simulink model "Jq_cc"  (R2015b)
settings: Solver=FixedStepDiscrete  StartTime=0.0  StopTime=0.01  FixedStep=0.010  RelTol=1e-3
PostLoadFcn:
  | , if any(exist('dsrtsu_mdlpostloadfcn', 'file') == [2, 3, 6]), try dsrtsu_mdlpostloadfcn('Execute', bdroot); catch fprintf('Error in PostLoadFcn (dsrtsu_mdlpostloadfcn) for model "%s":\n %s\n', bdroot, lasterr); end, end,
undefined symbols (not defined in the file or in its folder): DiscIntNeverNeededParam, lData
settings Model: DSRTSU_INTERNAL_RTI_VER=440  DSRTSU_INTERNAL_RTI_TYPE=rti1007  DSRTSU_INTERNAL_RTIFPGA=30  Creator=Mahl  LastModifiedBy=Mayer
settings DataIOCC: SaveFormat=Array
settings OptimizationCC: BlockReduction=off  OptimizeBlockIOStorage=off  BufferReuse=off  GlobalBufferReuse=off  ExpressionFolding=off  ExpressionDepthLimit=2147483647  LocalBlockOutputs=off
settings DebuggingCC: SolverPrmCheckMsg=warning  StateNameClashWarn=warning
settings HardwareCC: ProdBitPerPointer=32  ProdLargestAtomicFloat=None  ProdEndianess=BigEndian  ProdWordSize=32  ProdHWDeviceType=Generic->Custom  TargetIntDivRoundTo=Zero  TargetEndianess=BigEndian  TargetHWDeviceType=Generic->Custom
settings RTWCC: SystemTargetFile=rti1103.tlc  MakeCommand=make_rti  TemplateMakefile=rti1103.tmf  Description=dSPACE DS1103 Hardware Platform
settings STFCustomTargetCC: ParMdlRefBuildCompliant=on  ConcurrentExecutionCompliant=off  MatFileLogging=on  SystemTargetFile=rti1103.tlc
settings GRTTargetCC: CompOptLevelCompliant=off  ConcurrentExecutionCompliant=off  GeneratePreprocessorConditionals=Disable all  CombineOutputUpdateFcns=off  GRTInterface=on  UseToolchainInfoCompliant=off  ExtModeMexFile=noextcomm
settings ConfigComp: CovModelRefEnable=Off

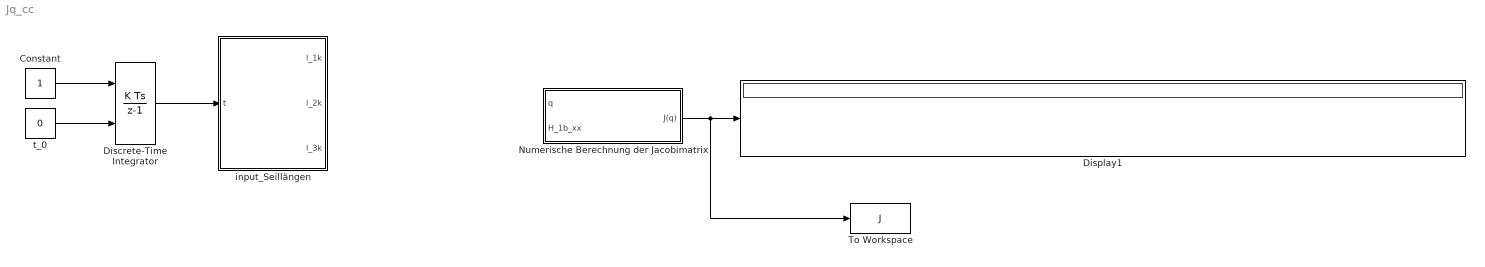
== system Jq_cc ==
  Constant : Constant
  Discrete-Time Integrator : DiscreteIntegrator  InitialConditionSource=external  InitialConditionSetting=State (most efficient)  SampleTime=0.010  ICPrevOutput=DiscIntNeverNeededParam  ICPrevScaledInput=DiscIntNeverNeededParam
  Display1 : Display
  Numerische Berechnung der Jacobimatrix : Subsystem
  To Workspace : ToWorkspace  VariableName=J  SampleTime=-1
  input_Seillängen : Subsystem
  t_0 : Constant  Value=0
  wires:
  Discrete-Time Integrator/1 -> input_Seillängen/1(t)
  Constant/1 -> Discrete-Time Integrator/1
  t_0/1 -> Discrete-Time Integrator/2
  Numerische Berechnung der Jacobimatrix/1(J(q)) -> Display1/1, To Workspace/1

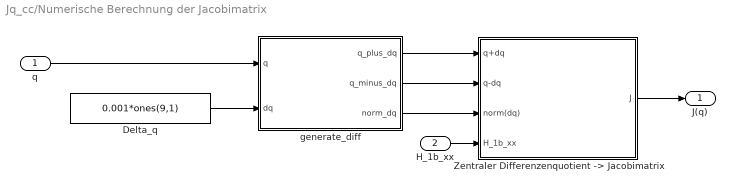
== system Jq_cc/Numerische Berechnung der Jacobimatrix ==
  q : Inport
  H_1b_xx : Inport  Port=2
  Delta_q : Constant  Value=0.001*ones(9,1)
  "Zentraler Differenzenquotient -> Jacobimatrix" : Subsystem  TreatAsAtomicUnit=on
  generate_diff : MATLAB Function  TreatAsAtomicUnit=on
  J(q) : Outport
  wires:
  H_1b_xx/1 -> "Zentraler Differenzenquotient -> Jacobimatrix"/4(H_1b_xx)
  Delta_q/1 -> generate_diff/2(dq)
  generate_diff/3(norm_dq) -> "Zentraler Differenzenquotient -> Jacobimatrix"/3(norm(dq))
  generate_diff/2(q_minus_dq) -> "Zentraler Differenzenquotient -> Jacobimatrix"/2(q-dq)
  generate_diff/1(q_plus_dq) -> "Zentraler Differenzenquotient -> Jacobimatrix"/1(q+dq)
  q/1 -> generate_diff/1(q)
  "Zentraler Differenzenquotient -> Jacobimatrix"/1(J) -> J(q)/1

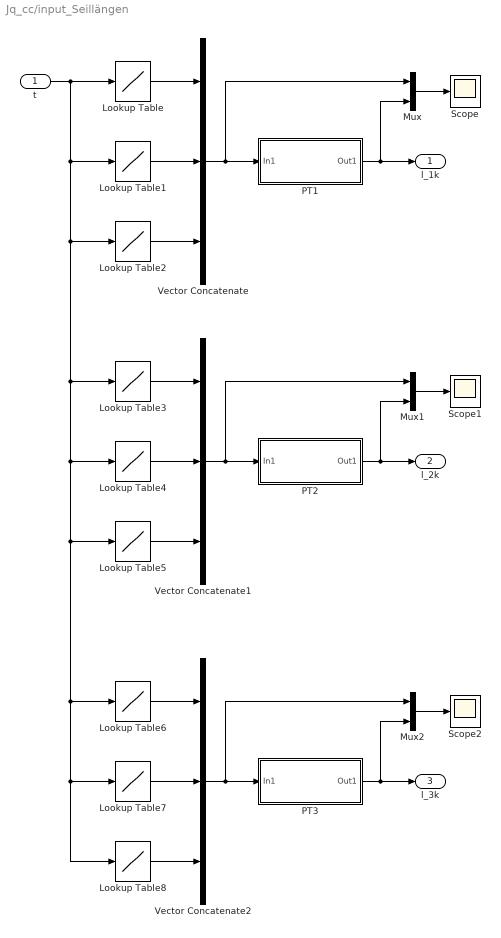
== system Jq_cc/input_Seillängen ==
  t : Inport
  Lookup Table : Lookup_n-D  NumberOfTableDimensions=1  BreakpointsForDimension1=lData.time  Table=lData.l_1k(1,:)  ExtrapMethod=Clip  InternalRulePriority=Speed  InputSameDT=on
      settings: AttributesFormatString=%<Table>
  Lookup Table1 : Lookup_n-D  NumberOfTableDimensions=1  BreakpointsForDimension1=lData.time  Table=lData.l_1k(2,:)  ExtrapMethod=Clip  InternalRulePriority=Speed  InputSameDT=on
      settings: AttributesFormatString=%<Table>
  Lookup Table2 : Lookup_n-D  NumberOfTableDimensions=1  BreakpointsForDimension1=lData.time  Table=lData.l_1k(3,:)  ExtrapMethod=Clip  InternalRulePriority=Speed  InputSameDT=on
      settings: AttributesFormatString=%<Table>
  Lookup Table3 : Lookup_n-D  NumberOfTableDimensions=1  BreakpointsForDimension1=lData.time  Table=lData.l_2k(1,:)  ExtrapMethod=Clip  InternalRulePriority=Speed  InputSameDT=on
      settings: AttributesFormatString=%<Table>
  Lookup Table4 : Lookup_n-D  NumberOfTableDimensions=1  BreakpointsForDimension1=lData.time  Table=lData.l_2k(2,:)  ExtrapMethod=Clip  InternalRulePriority=Speed  InputSameDT=on
      settings: AttributesFormatString=%<Table>
  Lookup Table5 : Lookup_n-D  NumberOfTableDimensions=1  BreakpointsForDimension1=lData.time  Table=lData.l_2k(3,:)  ExtrapMethod=Clip  InternalRulePriority=Speed  InputSameDT=on
      settings: AttributesFormatString=%<Table>
  Lookup Table6 : Lookup_n-D  NumberOfTableDimensions=1  BreakpointsForDimension1=lData.time  Table=lData.l_3k(1,:)  ExtrapMethod=Clip  InternalRulePriority=Speed  InputSameDT=on
      settings: AttributesFormatString=%<Table>
  Lookup Table7 : Lookup_n-D  NumberOfTableDimensions=1  BreakpointsForDimension1=lData.time  Table=lData.l_3k(2,:)  ExtrapMethod=Clip  InternalRulePriority=Speed  InputSameDT=on
      settings: AttributesFormatString=%<Table>
  Lookup Table8 : Lookup_n-D  NumberOfTableDimensions=1  BreakpointsForDimension1=lData.time  Table=lData.l_3k(3,:)  ExtrapMethod=Clip  InternalRulePriority=Speed  InputSameDT=on
      settings: AttributesFormatString=%<Table>
  Mux : Mux  Inputs=2
  Mux1 : Mux  Inputs=2
  Mux2 : Mux  Inputs=2
  PT1 : Subsystem
  PT2 : Subsystem
  PT3 : Subsystem
  Scope : Scope
  Scope1 : Scope
  Scope2 : Scope
  Vector Concatenate : Concatenate  NumInputs=3  Mode=Multidimensional array
  Vector Concatenate1 : Concatenate  NumInputs=3  Mode=Multidimensional array
  Vector Concatenate2 : Concatenate  NumInputs=3  Mode=Multidimensional array
  l_1k : Outport
  l_2k : Outport  Port=2
  l_3k : Outport  Port=3
  wires:
  t/1 -> Lookup Table1/1, Lookup Table2/1, Lookup Table3/1, Lookup Table4/1, Lookup Table5/1, Lookup Table6/1, Lookup Table7/1, Lookup Table8/1, Lookup Table/1
  Lookup Table/1 -> Vector Concatenate/1
  Lookup Table1/1 -> Vector Concatenate/2
  Lookup Table2/1 -> Vector Concatenate/3
  Vector Concatenate/1 -> PT1/1(In1), Mux/1
  PT1/1(Out1) -> l_1k/1, Mux/2
  Mux/1 -> Scope/1
  Lookup Table3/1 -> Vector Concatenate1/1
  Lookup Table4/1 -> Vector Concatenate1/2
  Lookup Table5/1 -> Vector Concatenate1/3
  Vector Concatenate1/1 -> Mux1/1, PT2/1(In1)
  PT2/1(Out1) -> Mux1/2, l_2k/1
  Mux1/1 -> Scope1/1
  Lookup Table6/1 -> Vector Concatenate2/1
  Lookup Table7/1 -> Vector Concatenate2/2
  Lookup Table8/1 -> Vector Concatenate2/3
  Vector Concatenate2/1 -> PT3/1(In1), Mux2/1
  PT3/1(Out1) -> l_3k/1, Mux2/2
  Mux2/1 -> Scope2/1

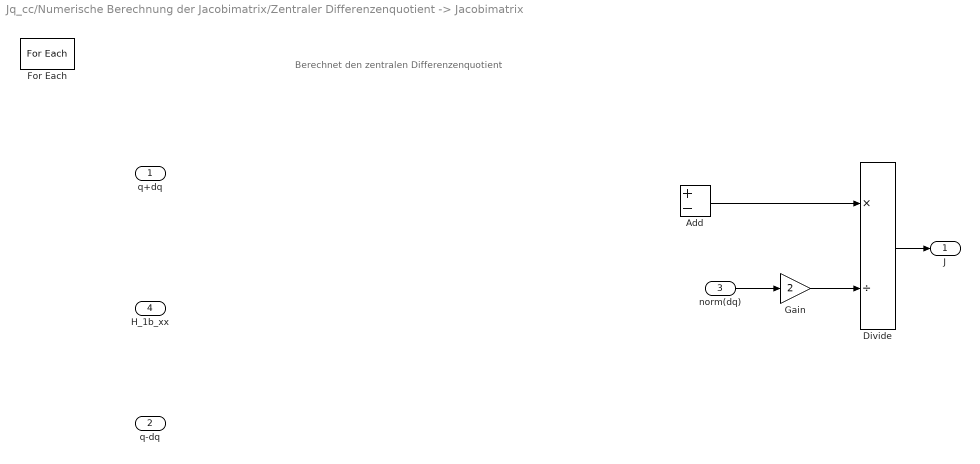
== system Jq_cc/Numerische Berechnung der Jacobimatrix/Zentraler Differenzenquotient -> Jacobimatrix ==
  note: Berechnet den zentralen Differenzenquotient
  q+dq : Inport  Partition=on  PartitionDimension=1  PartitionWidth=1
  q-dq : Inport  Port=2  Partition=on  PartitionDimension=1  PartitionWidth=1
  norm(dq) : Inport  Port=3  Partition=on  PartitionDimension=1  PartitionWidth=1
  H_1b_xx : Inport  Port=4
  Add : Sum  Inputs=+-
  Divide : Product  Inputs=*/
  For Each : ForEach  DisableCoverage=on  IndexMode=One-based
  Gain : Gain  Gain=2
  J : Outport  ConcatenationDimension=2
  wires:
  Gain/1 -> Divide/2
  Add/1 -> Divide/1
  Divide/1 -> J/1
  norm(dq)/1 -> Gain/1

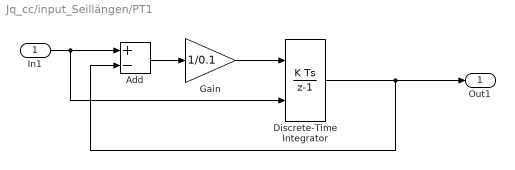
== system Jq_cc/input_Seillängen/PT1 ==
  In1 : Inport
  Add : Sum  Inputs=+-
  Discrete-Time Integrator : DiscreteIntegrator  InitialConditionSource=external  InitialConditionSetting=State (most efficient)  SampleTime=0.010  ICPrevOutput=DiscIntNeverNeededParam  ICPrevScaledInput=DiscIntNeverNeededParam
  Gain : Gain  Gain=1/0.1
  Out1 : Outport
  wires:
  In1/1 -> Add/1, Discrete-Time Integrator/2
  Add/1 -> Gain/1
  Discrete-Time Integrator/1 -> Out1/1, Add/2
  Gain/1 -> Discrete-Time Integrator/1

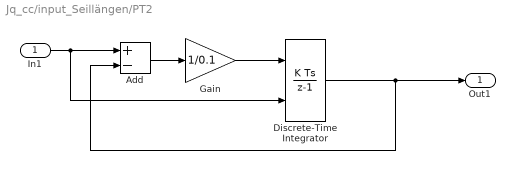
== system Jq_cc/input_Seillängen/PT2 ==
  In1 : Inport
  Add : Sum  Inputs=+-
  Discrete-Time Integrator : DiscreteIntegrator  InitialConditionSource=external  InitialConditionSetting=State (most efficient)  SampleTime=0.010  ICPrevOutput=DiscIntNeverNeededParam  ICPrevScaledInput=DiscIntNeverNeededParam
  Gain : Gain  Gain=1/0.1
  Out1 : Outport
  wires:
  Gain/1 -> Discrete-Time Integrator/1
  Discrete-Time Integrator/1 -> Add/2, Out1/1
  Add/1 -> Gain/1
  In1/1 -> Discrete-Time Integrator/2, Add/1

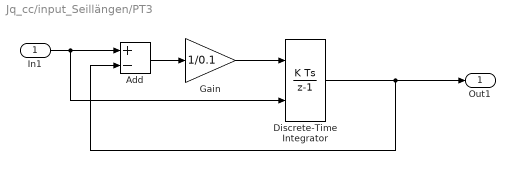
== system Jq_cc/input_Seillängen/PT3 ==
  In1 : Inport
  Add : Sum  Inputs=+-
  Discrete-Time Integrator : DiscreteIntegrator  InitialConditionSource=external  InitialConditionSetting=State (most efficient)  SampleTime=0.010  ICPrevOutput=DiscIntNeverNeededParam  ICPrevScaledInput=DiscIntNeverNeededParam
  Gain : Gain  Gain=1/0.1
  Out1 : Outport
  wires:
  In1/1 -> Add/1, Discrete-Time Integrator/2
  Add/1 -> Gain/1
  Discrete-Time Integrator/1 -> Out1/1, Add/2
  Gain/1 -> Discrete-Time Integrator/1

== matlab function Jq_cc/Numerische Berechnung der Jacobimatrix/generate_diff ==
  data: q input size=[9,1]; q_plus_dq output size=[9,1,9]; dq input size=[9,1]; q_minus_dq output size=[9,1,9]; norm_dq output size=[1,1,9]
function [q_plus_dq, q_minus_dq, norm_dq] = gen_diff(q, dq)
% Input:
% q     [nx1]   Zustand Gelenkvariablen
% dq    [nx1]   Betrag der differentiellen Aenderung je Gelenkzustand zur
%               Ableitungsbestimmung (->Jacobimatrix)
%
% Output:
% qpdq  [nx1xn] Gelenkzustand zuzüglich diferentieller Änderung
%               Reihenfolge: nx1x1 = [q1+dq1; q2; ...; qn]
%                            nx1x2 = [q1; q2+dq2; ...; qn] 
%                                  : 
%                            nx1xn = [q1; q2; ...; qn+dqn]
% qmdq  [nx1xn] Gelenkzustand abzüglich diferentieller Änderung
%               Reihenfolge: nx1x1 = [q1-dq1; q2; ...; qn]
%                            nx1x2 = [q1; q2-dq2; ...; qn] 
%                                  : 
%                            nx1xn = [q1; q2; ...; qn-dqn] 
% ndq   [1x1xn] Norm der differentiellen Änderung

n               = 9;
q_plus_dq       = zeros(n,1,n);
q_minus_dq      = zeros(n,1,n);
norm_dq         = zeros(1,1,n);

norm_dq(1,1,:)  = ;
q_plus_dq = 
q_minus_dq =
